simulink model "model_z_obserwatorem"  (R2017b)
settings: Solver=VariableStepAuto  StartTime=0.0  StopTime=10.0  RelTol=1e-3
values from neighbouring files (symbols this model uses):
  a11 = A2(1,1)    [pkt10.m]    (also in pkt9.m)
  A2 = A1'    [initial_values.m]    (also in matlab.mat = [3.22791678547  1  0; -1.44925930399  0  1; 0.17377394345  0)
  a21 = A2(2,1)    [pkt10.m]    (also in pkt9.m)
  a31 = A2(3,1)    [pkt10.m]    (also in pkt9.m)
  b1 = B2(1)    [pkt10.m]    (also in pkt9.m)
  B2 = C1'    [initial_values.m]    (also in matlab.mat = [0.260707487539 -0.289205764977 0.0761198486843])
  b2 = B2(2)    [pkt10.m]    (also in pkt9.m)
  b3 = B2(3)    [pkt10.m]    (also in pkt9.m)
  K = [-150 -150 -150]    [matlab.mat]    (also in pkt10.m = acker(A2,B2,[0.25,0.2+0.1i,-0.1i]); pkt6rzeczywiste.m = acker(A2,B2,[pole,pole,pole]); pkt6zespolone.m = acker(A2,B2,[zb1,zb2,zb3]); pkt7.m = Kpol(iter,:))
  l1 = L(1)    [pkt10.m]    (also in pkt9.m)
  l2 = L(2)    [pkt10.m]    (also in pkt9.m)
  Tp = 0.25    [initial_values.m]    (also in matlab.mat)
  X0 = [8 2 -1]    [pkt10.m]    (also in pkt6rzeczywiste.m; pkt6zespolone.m; pkt7.m; pkt7best.m)
settings Model: Creator=Paweł  LastModifiedBy=Paweł

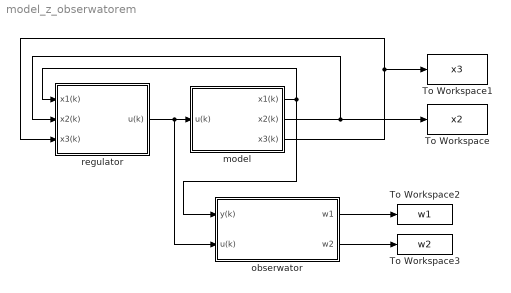
== system model_z_obserwatorem ==
  To Workspace : ToWorkspace  VariableName=x2  SaveFormat=Timeseries  SampleTime=-1
  To Workspace1 : ToWorkspace  VariableName=x3  SaveFormat=Timeseries  SampleTime=-1
  To Workspace2 : ToWorkspace  VariableName=w1  SaveFormat=Timeseries  SampleTime=-1
  To Workspace3 : ToWorkspace  VariableName=w2  SaveFormat=Timeseries  SampleTime=-1
  model : Subsystem
  obserwator : Subsystem
  regulator : Subsystem
  wires:
  model/3(x3(k)) -> regulator/3(x3(k)), To Workspace1/1
  obserwator/1(w1) -> To Workspace2/1
  regulator/1("u(k) ") -> obserwator/2(u(k)), model/1("u(k) ")
  obserwator/2(w2) -> To Workspace3/1
  model/2(x2(k)) -> regulator/2(x2(k)), To Workspace/1
  model/1(x1(k)) -> obserwator/1(y(k)), regulator/1(x1(k))

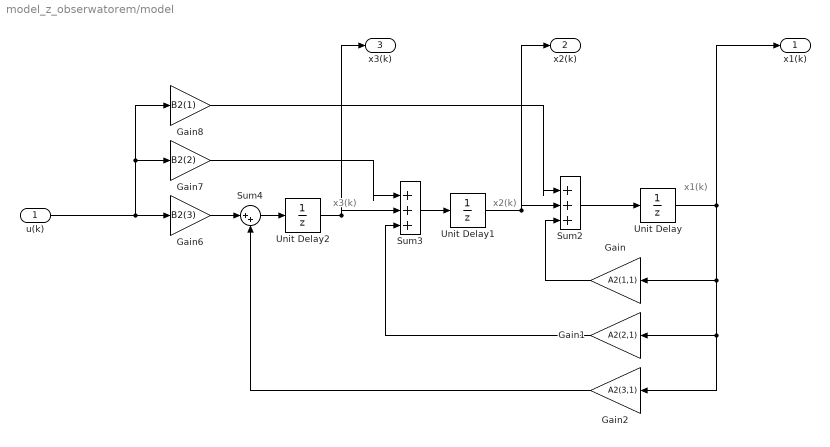
== system model_z_obserwatorem/model ==
  note: x1(k)
  note: x3(k)
  note: x2(k)
  "u(k) " : Inport
  Gain : Gain  Gain=A2(1,1)
  Gain1 : Gain  Gain=A2(2,1)
  Gain2 : Gain  Gain=A2(3,1)
  Gain6 : Gain  Gain=B2(3)
  Gain7 : Gain  Gain=B2(2)
  Gain8 : Gain  Gain=B2(1)
  Sum2 : Sum  Inputs=|+++
  Sum3 : Sum  Inputs=|+++
  Sum4 : Sum  Inputs=|++
  Unit Delay : UnitDelay  InitialCondition=X0(1)  SampleTime=Tp
  Unit Delay1 : UnitDelay  InitialCondition=X0(2)  SampleTime=Tp
  Unit Delay2 : UnitDelay  InitialCondition=X0(3)  SampleTime=Tp
  x1(k) : Outport
  x2(k) : Outport  Port=2
  x3(k) : Outport  Port=3
  wires:
  Sum3/1 -> Unit Delay1/1
  Gain/1 -> Sum2/3
  Sum4/1 -> Unit Delay2/1
  Gain6/1 -> Sum4/1
  Gain7/1 -> Sum3/1
  Gain8/1 -> Sum2/1
  "u(k) "/1 -> Gain8/1, Gain7/1, Gain6/1
  Gain1/1 -> Sum3/3
  Unit Delay1/1 -> x2(k)/1, Sum2/2
  Unit Delay/1 -> Gain2/1, Gain1/1, Gain/1, x1(k)/1
  Gain2/1 -> Sum4/2
  Sum2/1 -> Unit Delay/1
  Unit Delay2/1 -> Sum3/2, x3(k)/1

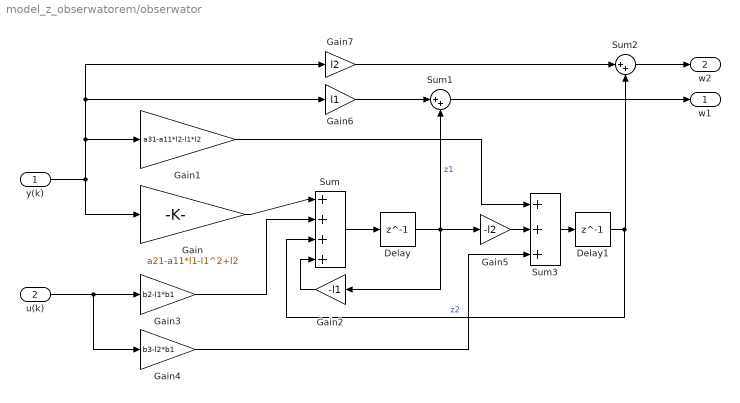
== system model_z_obserwatorem/obserwator ==
  y(k) : Inport
  u(k) : Inport  Port=2
  Delay : Delay  DelayLength=1  SampleTime=Tp
  Delay1 : Delay  DelayLength=1  SampleTime=Tp
  Gain : Gain  Gain=a21-a11*l1-l1^2+l2
  Gain1 : Gain  Gain=a31-a11*l2-l1*l2
  Gain2 : Gain  Gain=-l1
  Gain3 : Gain  Gain=b2-l1*b1
  Gain4 : Gain  Gain=b3-l2*b1
  Gain5 : Gain  Gain=-l2
  Gain6 : Gain  Gain=l1
  Gain7 : Gain  Gain=l2
  Sum : Sum  Inputs=|++++
  Sum1 : Sum  Inputs=|++
  Sum2 : Sum  Inputs=|++
  Sum3 : Sum  Inputs=+++
  w1 : Outport
  w2 : Outport  Port=2
  wires:
  Sum/1 -> Delay/1
  Sum3/1 -> Delay1/1
  y(k)/1 -> Gain7/1, Gain6/1, Gain1/1, Gain/1
  Delay/1 -> Gain2/1, Sum1/2, Gain5/1  "z1"
  Gain/1 -> Sum/1
  Gain2/1 -> Sum/4
  Delay1/1 -> Sum2/2, Sum/3  "z2"
  u(k)/1 -> Gain4/1, Gain3/1
  Gain3/1 -> Sum/2
  Gain4/1 -> Sum3/3
  Gain1/1 -> Sum3/1
  Gain5/1 -> Sum3/2
  Gain6/1 -> Sum1/1
  Sum1/1 -> w1/1
  Gain7/1 -> Sum2/1
  Sum2/1 -> w2/1

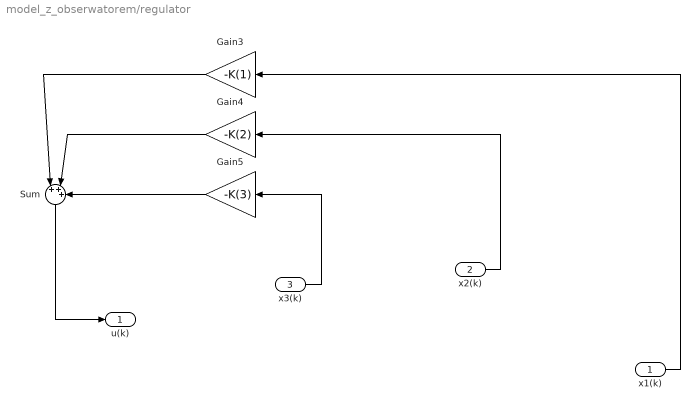
== system model_z_obserwatorem/regulator ==
  x1(k) : Inport
  x2(k) : Inport  Port=2
  x3(k) : Inport  Port=3
  Gain3 : Gain  Gain=-K(1)
  Gain4 : Gain  Gain=-K(2)
  Gain5 : Gain  Gain=-K(3)
  Sum : Sum  Inputs=|+++
  "u(k) " : Outport
  wires:
  Sum/1 -> "u(k) "/1
  x1(k)/1 -> Gain3/1
  x3(k)/1 -> Gain5/1
  x2(k)/1 -> Gain4/1
  Gain5/1 -> Sum/3
  Gain4/1 -> Sum/2
  Gain3/1 -> Sum/1
